simulink model "PID_vehicle"  (R2021a)
settings: Solver=VariableStepAuto  StartTime=0.0  StopTime=sim_time  MaxStep=step_value  RelTol=1e-3
values from neighbouring files (symbols this model uses):
  b = 3.5077E-6    (= 3.5077e-06)    [DCMotor_reduction_run.m]    (also in DCMotor_run.m; MassSpringDamper_run.m = 2; PID_ScriptOnly.m = 50; PID_SpringDamper_run.m = 10)
  Kd = 0    [DCMotor_reduction_run.m]    (also in PID_SpringDamper_run.m = 50; PID_block_run.m; PID_vehicle_run.m)
  Ki = 1    [DCMotor_reduction_run.m]    (also in PID_ScriptOnly.m = 40; PID_SpringDamper_run.m = 300; PID_block_run.m = 0; PID_vehicle_run.m)
  Kp = 0.5    [DCMotor_reduction_run.m]    (also in PID_ScriptOnly.m = 800; PID_SpringDamper_run.m = 350; PID_block_run.m = 1000; PID_vehicle_run.m = 1)
  M = 1    [MassSpringDamper_run.m]    (also in PID_SpringDamper_run.m; PID_block_run.m; PID_vehicle_run.m; TransferFunctionModel_run.m)
  step_final = 10    [PID_block_run.m]    (also in PID_vehicle_run.m)
libraries: pid_lib x1
settings Model: Creator=shinyh  LastModifiedBy=shinyh

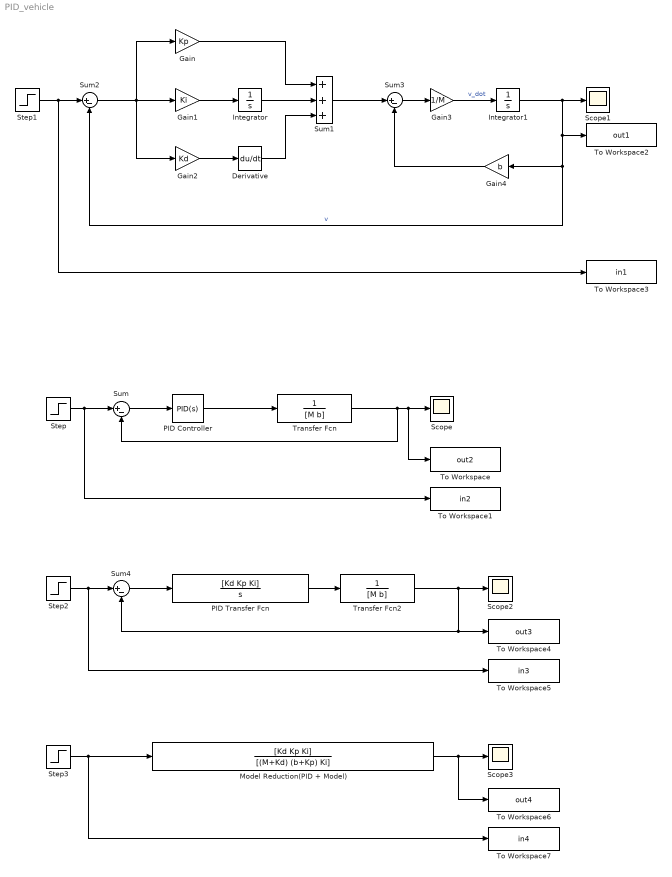
== system PID_vehicle ==
  Derivative : Derivative
  Gain : Gain  Gain=Kp
  Gain1 : Gain  Gain=Ki
  Gain2 : Gain  Gain=Kd
  Gain3 : Gain  Gain=1/M
  Gain4 : Gain  Gain=b
  Integrator : Integrator
  Integrator1 : Integrator
  Model Reduction(PID + Model) : TransferFcn  Numerator=[Kd Kp Ki]  Denominator=[(M+Kd) (b+Kp) Ki]
  PID Controller : pid_lib/PID Controller  Controller=PID  Form=Parallel  TimeDomain=Continuous-time  UseExternalTs=off  SampleTime=-1  IntegratorMethod=Forward Euler  FilterMethod=Forward Euler  ControllerParametersSource=internal  P=Kp  I=Ki  D=Kd  UseFilter=on  N=1367.57064052508  TunerSelectOption=Transfer Function Based (PID Tuner App)  InitialConditionSource=internal  InitialConditionForIntegrator=0  InitialConditionForFilter=0  DifferentiatorICPrevScaledInput=0  ExternalReset=none  TrackingMode=off  Kt=1  LimitOutput=off  SatLimitsSource=internal  UpperSaturationLimit=inf  LowerSaturationLimit=-inf  LinearizeAsGain=on  AntiWindupMode=none  Kb=1  POutMin=[]  POutMax=[]  IOutMin=[]  IOutMax=[]  DOutMin=[]  DOutMax=[]  NOutMin=[]  NOutMax=[]  SumOutMin=[]  SumOutMax=[]  SaturationOutMin=[]  SaturationOutMax=[]  PParamMin=[]  PParamMax=[]  IParamMin=[]  IParamMax=[]  DParamMin=[]  DParamMax=[]  NParamMin=[]  NParamMax=[]  KbParamMin=[]  KbParamMax=[]  KtParamMin=[]  KtParamMax=[]  KbOutMin=[]  KbOutMax=[]  KtOutMin=[]  KtOutMax=[]  IntegratorOutMin=[]  IntegratorOutMax=[]  FilterOutMin=[]  FilterOutMax=[]  SumI1OutMin=[]  SumI1OutMax=[]  SumI2OutMin=[]  SumI2OutMax=[]  SumI3OutMin=[]  SumI3OutMax=[]  SumI4OutMin=[]  SumI4OutMax=[]  SumDOutMin=[]  SumDOutMax=[]  DifferentiatorOutMin=[]  DifferentiatorOutMax=[]  FilterDiffOutCoefMin=[]  FilterDiffOutCoefMax=[]  ReciprocalOutMin=[]  ReciprocalOutMax=[]  SumDenOutMin=[]  SumDenOutMax=[]  SumNumOutMin=[]  SumNumOutMax=[]  DivideOutMin=[]  DivideOutMax=[]  UdiffTsProdOutMin=[]  UdiffTsProdOutMax=[]  NTsProdOutMin=[]  NTsProdOutMax=[]  UintegralTsProdOutMin=[]  UintegralTsProdOutMax=[]  UngainTsProdOutMin=[]  UngainTsProdOutMax=[]  IntegratorContinuousStateAttributes=''  IntegratorStateMustResolveToSignalObject=off  IntegratorRTWStateStorageClass=Auto  FilterContinuousStateAttributes=''  FilterStateMustResolveToSignalObject=off  FilterRTWStateStorageClass=Auto  ParallelPVariant=InternalParameters  IdealPVariant=Disabled  IVariant=InternalParameters  DVariant=InternalParameters  IntegratorVariant=Continuous  SatVariant=Disabled  AWVariant=Passthrough  PCopyVariant=Disabled  TRVariant=Disabled  FdbkBlocksVariant=Forward  IdealPFdbkVariant=Disabled  SatFdbkVariant=Disabled  DerivativeFilterVariant=ContFilter  NVariant=InternalParameters  NCopyVariant=Disabled  FilterICVariant=InternalICsFilter  IntegratorICVariant=InternalICs  ExternalResetVariant=Disabled  TRSumVariant=Passthrough  SumFdbkVariant=Disabled  SumVariant=Sum_PID  TsampFilterVariant=InternalTs  TsampNgainVariant=Passthrough  TsampIntegralVariant=Passthrough  ExternalSaturationOutDataTypeStr=Inherit: Same as second input
  PID Transfer Fcn : TransferFcn  Numerator=[Kd Kp Ki]  Denominator=[1 0]
  Scope{,1..3} (4 alike) : Scope
  Step{,1..3} (4 alike) : Step  After=step_final  SampleTime=0
  Sum{,2..4} (4 alike) : Sum  Inputs=|+-
  Sum1 : Sum  Inputs=+++
  To Workspace : ToWorkspace  VariableName=out2  SaveFormat=Timeseries  SampleTime=-1
  To Workspace1 : ToWorkspace  VariableName=in2  SaveFormat=Timeseries  SampleTime=-1
  To Workspace2 : ToWorkspace  VariableName=out1  SaveFormat=Timeseries  SampleTime=-1
  To Workspace3 : ToWorkspace  VariableName=in1  SaveFormat=Timeseries  SampleTime=-1
  To Workspace4 : ToWorkspace  VariableName=out3  SaveFormat=Timeseries  SampleTime=-1
  To Workspace5 : ToWorkspace  VariableName=in3  SaveFormat=Timeseries  SampleTime=-1
  To Workspace6 : ToWorkspace  VariableName=out4  SaveFormat=Timeseries  SampleTime=-1
  To Workspace7 : ToWorkspace  VariableName=in4  SaveFormat=Timeseries  SampleTime=-1
  Transfer Fcn : TransferFcn  Denominator=[M b]
  Transfer Fcn2 : TransferFcn  Denominator=[M b]
  wires:
  PID Controller/1 -> Transfer Fcn/1
  Sum/1 -> PID Controller/1
  Transfer Fcn/1 -> To Workspace/1, Scope/1, Sum/2
  Step/1 -> To Workspace1/1, Sum/1
  Derivative/1 -> Sum1/3
  Sum1/1 -> Sum3/1
  Gain/1 -> Sum1/1
  Gain1/1 -> Integrator/1
  Integrator/1 -> Sum1/2
  Gain2/1 -> Derivative/1
  Gain3/1 -> Integrator1/1  "v_dot"
  Integrator1/1 -> Scope1/1, Gain4/1, Sum2/2, To Workspace2/1  "v"
  Gain4/1 -> Sum3/2
  Sum3/1 -> Gain3/1
  Sum2/1 -> Gain2/1, Gain1/1, Gain/1
  Step1/1 -> To Workspace3/1, Sum2/1
  Step2/1 -> To Workspace5/1, Sum4/1
  Sum4/1 -> PID Transfer Fcn/1
  PID Transfer Fcn/1 -> Transfer Fcn2/1
  Transfer Fcn2/1 -> Sum4/2, To Workspace4/1, Scope2/1
  Model Reduction(PID + Model)/1 -> Scope3/1, To Workspace6/1
  Step3/1 -> Model Reduction(PID + Model)/1, To Workspace7/1
